simulink model "TBRe19_ECU_PW_Testbench"  (R2017b)
settings: Solver=FixedStepDiscrete  StartTime=0.0  StopTime=inf  FixedStep=0.0001  RelTol=1e-3
PostLoadFcn:
  | model_init();
libraries: simulink_extras x1
(part 1 of 5)
settings Model: Creator=agf25  LastModifiedBy=Peter
settings DataIOCC: LimitDataPoints=on
settings OptimizationCC: DefaultParameterBehavior=Inlined  EfficientFloat2IntCast=on  LifeSpan=inf
settings DebuggingCC: AllowSymbolicDim=off  SFUnexpectedBacktrackingDiag=warning  SFNoUnconditionalDefaultTransitionDiag=warning  SFExecutionAtInitializationDiag=none
settings ModelReferenceCC: PropagateSignalLabelsOutOfModel=off
settings RTWCC: SystemTargetFile=nsi_mpc.tlc  MakeCommand=nsi_make  TemplateMakefile=nsi_mpc.tmf  Description=RTW Coder for MUXLAB4
settings CodeAppCC: StateflowObjectComments=on
settings STFCustomTargetCC: MATLABClassNameForMDSCustomization=Simulink.SoftwareTarget.TargetSpecificTriggerConfigurationBase  SystemTargetFile=nsi_mpc.tlc
settings ConfigComp: CovMetricSettings=dw  CovHtmlReporting=on  CovSaveCumulativeToWorkspaceVar=on  CovSaveSingleToWorkspaceVar=on  CovExternalEMLEnable=off
settings SimscapeCC: SimscapeNormalizeSystem=off
settings ConfigurationSet: Description=SimMechanics 2G

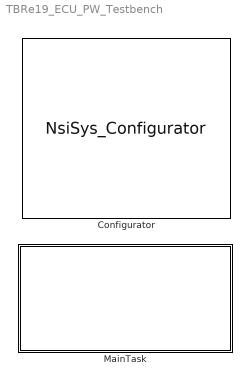
== system TBRe19_ECU_PW_Testbench ==
  Configurator : S-Function  FunctionName=NsiSys_Configurator  Parameters=main,io,nbof_can,can,ccp,flash,nbof_lin,lin,tasks  SFunctionDeploymentMode=off  EnableBusSupport=off  mask(Configurator block){main=Config description;01/01/2011;0;0.000000, io=2.5;0;1;1;1;1;1;1;1, nbof_can=5, can=1;HIGH_SPEED;500Kbps;No;C:\Users\Peter\Google_Drive\Year_5\TBRe\03-Design_Files\ECU\ECU-Model\TBRe19_DBC.dbc;0;1;1Mbits;0;HIGH_SPEED;500Kbps;120 Ohm;C:\Users\TBRe-admin\Documents\Database\TBRe19_DBC_190517.dbc;0;0;1Mbits;0;HIGH_SPEED;1000Kbps;120 Ohm;D:\TOOLS\MUXLINK\R2011b\MUXlink\misc\BASE_CAN_MUXLAB4.dbc;0;0;1Mbits;0;HIGH_SPEED;500Kbps;120 Ohm;D:\TOOLS\MUXLINK\R2011b\MUXlink\misc\j1939_adapt.dbc;0;1;1Mbits;0;HIGH_SPEED;1000Kbps;No;D:\TOOLS\MUXLINK\R2011b\MUXlink\misc\BASE_CAN_MUXLAB4.dbc;0;0;1Mbits, ccp=2;0x100;0x200;0;0;0x0;0x0;0;0x13, flash=, nbof_lin=2, lin=0;D:\TOOLS\MUXLINK\R2011b\MUXlink\misc\lindb.ldf;1;0.0;0.0;0.000;0.000;0.000000;0,0;0;D:\TOOLS\MUXLINK\R2011b\MUXlink\misc\lindb.ldf;1;0.0;0.0;0.000;0.000;0.000000;0,0, tasks=MainTask;[0.01]}
      mask prompts: nbof_can "nbof can"
      mask help: This block permits to set general parameters to use a MUXlink model
      mask init:
      | NsiSys_Configurator_InitializationFcn();
      settings: OpenFcn=NsiSys_Configurator_OpenFcn();
      mask Help:
      | eval('block=get_param(gcb, ''RTWdata'');')
      | web([docroot '\toolbox\MUXlink\html\blocks/' block.MUXlink_BlockType '.html'])
      mask Callback main: NsiSys_Configurator_ApplyFcn(1);
      mask Callback io: NsiSys_Configurator_ApplyFcn(2);
      mask Callback nbof_can: NsiSys_Configurator_ApplyFcn(3);
      mask Callback can: NsiSys_Configurator_ApplyFcn(4);
      mask Callback ccp: NsiSys_Configurator_ApplyFcn(5);
      mask Callback flash: NsiSys_Configurator_ApplyFcn(6);
      mask Callback nbof_lin: NsiSys_Configurator_ApplyFcn(7);
      mask Callback lin: NsiSys_Configurator_ApplyFcn(8);
      mask Callback tasks: NsiSys_Configurator_ApplyFcn(9);
      mask Display: image(imread('MUXLAB4.bmp'));text(0.5, 0.2, '', 'horizontalAlignment', 'center', 'verticalAlignment', 'base');
  MainTask : Subsystem  TreatAsAtomicUnit=on  SystemSampleTime=[0.01]  RTWFcnName=MainTask  RTWFileName=FileTaskFcn
      mask init:
      | NsiSys_SubSystemTask_InitializationFcn();
      settings: OpenFcn=NsiSys_SubSystemTask_OpenFcn();  RTWSystemCode=Nonreusable function  RTWFcnNameOpts=User specified  RTWFileNameOpts=Use function name
      mask Display: image(imread('nsi.bmp'));text(0.45, 0.9, 'task()');plot([0.05 0.05 0.05 0.05 0.05 0.05 0.05 0.05 0.05 0.05]);fprintf('MainTask\n/ 10.0ms / 0.0ms /\nEvent');

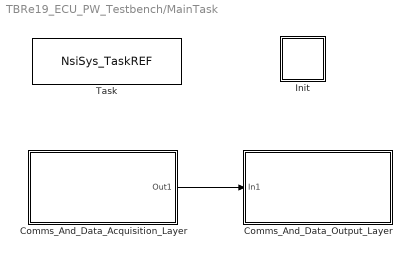
== system TBRe19_ECU_PW_Testbench/MainTask ==
  Comms_And_Data_Acquisition_Layer : Subsystem
  Comms_And_Data_Output_Layer : Subsystem
  Init : Subsystem  mask(System Initialize){}
      mask help: Add code to a systems Initialize function
      settings: CopyFcn=cccopyfcn(gcb)  OpenFcn=ccopenfcn('System Initialize Function')
      mask Help: This block contains text fields to insert custom user code sections at the declaration, execution and exit sections of the systems initialize function.  By placing this block inside a subsytem, the custom user code will appear in that subsystems function.
      mask Display: disp('I()')
  Task : S-Function  FunctionName=NsiSys_TaskREF  Parameters=task_initialised,task_periodic, task_sampletime,task_name,task_event,task_offset  SFunctionDeploymentMode=off  EnableBusSupport=off  mask(task definition){task_initialised=on, task_periodic=on, task_sampletime=[0.01], task_offset=0.00, task_name=MainTask, task_event=on}
      mask prompts: task_initialised "task initialised"; task_periodic "Is Periodic"; task_sampletime "Task sample time"; task_offset "Task Offset"; task_name "Task name"; task_event "Is event"
      mask help:
      | Permit to provide all parameters associated to a MUXLINK task.
      | Task can be executed periodicaly and/or on event detection.
      | If task is periodic:
      | Task sample time specify the execution period in mS [0.001   6000]
      | Task Offset specify the offset applied to the execution period
      | Task Offset < Task sample time
      mask init:
      | NsiSys_TaskREF_InitializationFcn();
      settings: OpenFcn=NsiSys_Task_OpenFcn();
      mask Callback task_initialised: NsiSys_TaskREF_ApplyFcn(1);
      mask Callback task_periodic: NsiSys_TaskREF_ApplyFcn(2);
      mask Callback task_sampletime: NsiSys_TaskREF_ApplyFcn(3);
      mask Callback task_offset: NsiSys_TaskREF_ApplyFcn(6);
      mask Callback task_name: NsiSys_TaskREF_ApplyFcn(4);
      mask Callback task_event: NsiSys_TaskREF_ApplyFcn(5);
      mask Display: text(0.5, 0.8, 't()', 'horizontalAlignment', 'center', 'verticalAlignment', 'base');text(0.5, 0.2, '/ 10.0ms / 0.0ms /', 'horizontalAlignment', 'center', 'verticalAlignment', 'base');text(0.5, 0.4, 'Event', 'horizontalAlignment', 'center', 'verticalAlignment', 'base');
  wires:
  Comms_And_Data_Acquisition_Layer/1(Out1) -> Comms_And_Data_Output_Layer/1(In1)

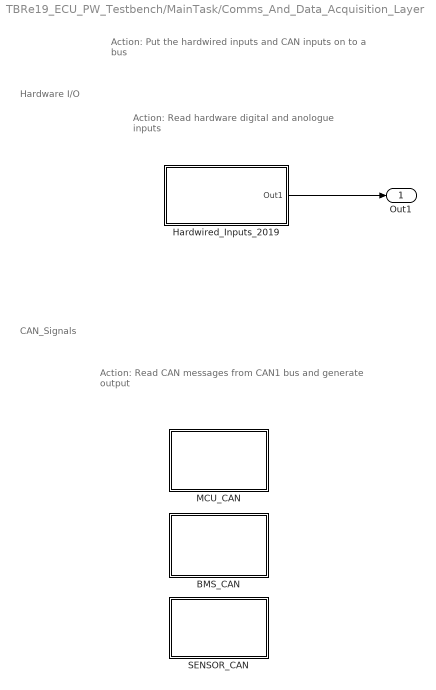
== system TBRe19_ECU_PW_Testbench/MainTask/Comms_And_Data_Acquisition_Layer ==
  note: Hardware I/O
  note: CAN_Signals
  note: Action:
      | Put the hardwired inputs and CAN inputs on to a bus
  note: Action:
      | Read CAN messages from CAN1 bus and generate output
  note: Action:
      | Read hardware digital and anologue inputs
  BMS_CAN : Subsystem
  Hardwired_Inputs_2019 : Subsystem
  MCU_CAN : Subsystem
  SENSOR_CAN : Subsystem
  Out1 : Outport
  wires:
  Hardwired_Inputs_2019/1(Out1) -> Out1/1
